simulink model "simulink_msd"  (R2018a)
settings: Solver=VariableStepAuto  StartTime=0.0  StopTime=20  RelTol=1e-3
settings Model: Creator=Arnab Banerjee  LastModifiedBy=Arnab Banerjee

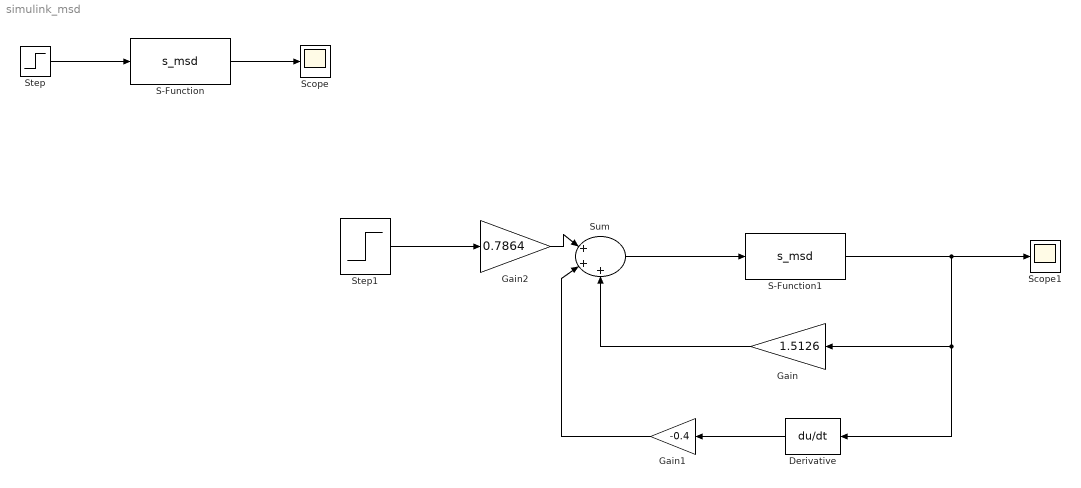
== system simulink_msd ==
  Derivative : Derivative
  Gain : Gain  Gain=1.5126
  Gain1 : Gain  Gain=-0.4
  Gain2 : Gain  Gain=0.7864
  S-Function : S-Function  FunctionName=s_msd  SFunctionDeploymentMode=off  EnableBusSupport=off
  S-Function1 : S-Function  FunctionName=s_msd  SFunctionDeploymentMode=off  EnableBusSupport=off
  Scope : Scope
  Scope1 : Scope
  Step : Step  Time=0  SampleTime=0
  Step1 : Step  Time=0  SampleTime=0
  Sum : Sum  Inputs=|+++
  wires:
  Step/1 -> S-Function/1
  S-Function/1 -> Scope/1
  Gain/1 -> Sum/3
  S-Function1/1 -> Derivative/1, Gain/1, Scope1/1
  Derivative/1 -> Gain1/1
  Gain1/1 -> Sum/2
  Sum/1 -> S-Function1/1
  Step1/1 -> Gain2/1
  Gain2/1 -> Sum/1
